simulink model "distmodelR2019a"  (R2020b)
settings: Solver=FixedStepAuto  StartTime=0.0  StopTime=t_sim  FixedStep=TimeStep  RelTol=1e-3
values from neighbouring files (symbols this model uses):
  alt = 300    [main_disturbances_Z.m]
  AX = 0.022    [calctorque.m]    (also in main_disturbances_Z.m)
  AY = 0.034    [calctorque.m]    (also in main_disturbances_Z.m)
  AZ = 0.0748    [calctorque.m]    (also in main_disturbances_Z.m = 0.2108)
  AZES = 0.1156    [calctorque.m]    (also in main_disturbances_Z.m)
  Cdrag = 2.6    [disturbanceCode.m]    (also in main_disturbances_Z.m)
  CLS = [0,-0.195,0.05]    [calctorque.m]    (also in main_disturbances_Z.m)
  Cmy = [0,-0.11,0]    [calctorque.m]    (also in main_disturbances_Z.m)
  CRS = [0,0.195,0.05]    [calctorque.m]    (also in main_disturbances_Z.m)
  D = [-0.17,0.11,0.05]    [projectionTorque1.m]    (also in projectionTorque2.m; projectionTorque3.m = [-0.17,-0.11,0.05]; projectionTorque4.m = [-0.17,-0.11,0.05])
  ESS = 0.0578    [calctorque.m]    (also in main_disturbances_Z.m)
  G = [OGX,OGY,OGZ]    [disturbanceCode.m]    (also in main_disturbances_Z.m)
  inc = rad2deg(inc)    [main_disturbances_Z.m]
  nu = rad2deg(nu)    [main_disturbances_Z.m]
  OGX = 2.5*1e-3    (= 0.0025)    [disturbanceCode.m]    (also in main_disturbances_Z.m = 0.00025)
  OGY = 1*1e-2    (= 0.01)    [disturbanceCode.m]    (also in main_disturbances_Z.m = -0.001)
  OGZ = 1*1e-2    (= 0.01)    [disturbanceCode.m]    (also in main_disturbances_Z.m = -0.002)
  OX = 0.17    [calctorque.m]    (also in main_disturbances_Z.m)
  OY = 0.11    [calctorque.m]    (also in main_disturbances_Z.m)
  OZ = 0.05    [calctorque.m]    (also in main_disturbances_Z.m)
  RAAN = rad2deg(RAAN)    [main_disturbances_Z.m]
  RSD = [0.08,0.08,0.08]    [main_disturbances_Z.m]
  w = rad2deg(w)    [main_disturbances_Z.m]
undefined symbols (not defined in the file or in its folder): date, DipoleMod, ecc, km, nmax, s, Use_IGRF
libraries: vrlib x19, dspmathops x6, sharedtransform x4, aerolibutil x4, dspindex x3, aerolibconvert2 x2, simulink_extras x1, aerolibatmos2 x1, aerolibcelestial x1, sharedutil x1, aerolibobsolete x1
(part 1 of 2)
settings Model: Creator=colpari  LastModifiedBy=colpari
settings SFSimCC: CustomCodeUndefinedFunction=UseInterfaceOnly

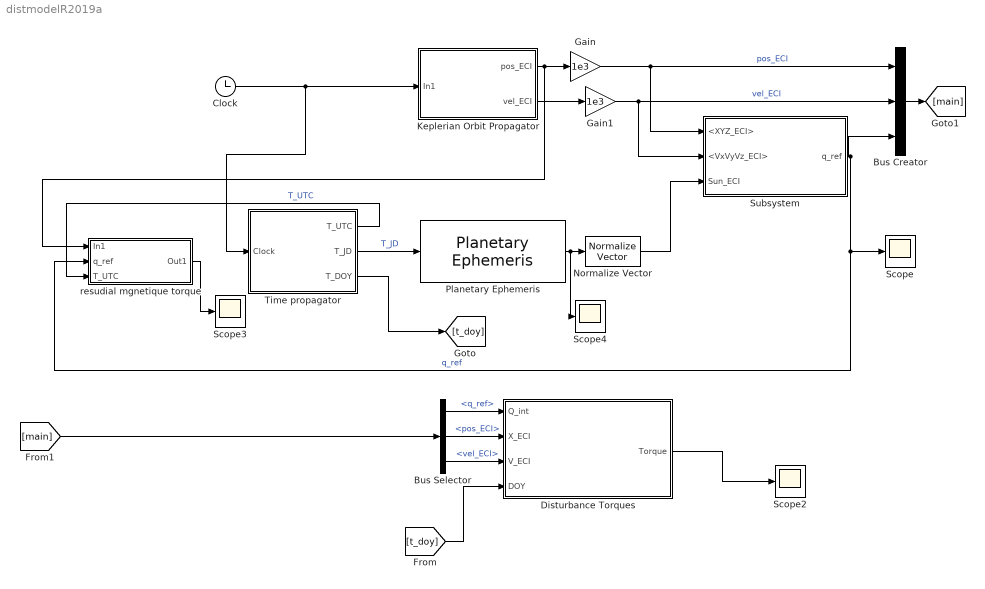
== system distmodelR2019a ==
  Bus Creator : BusCreator  Inputs=3
  Bus Selector : BusSelector  OutputSignals=q_ref,pos_ECI,vel_ECI
  Clock : Clock
  "Disturbance Torques " : Subsystem
  Gain : Gain  Gain=1e3
  Gain1 : Gain  Gain=1e3
  Keplerian Orbit Propagator : Subsystem
  Normalize Vector : vrlib/Utilities/Normalize Vector  maxzero=0
  Planetary Ephemeris : aerolibcelestial/Planetary Ephemeris  kmflag=km,km/s  epochflag=Julian date  de=DE405  nCenter=Earth  nTarget=Sun  errorflag=Error  velflag=off
      settings: SourceProductBaseCode=AE
  Scope{,2..4} (4 alike) : Scope
  Subsystem : Subsystem
  Time propagator : Subsystem
  "resudial mgnetique torque " : Subsystem
  wires:
  [t_doy] -> "Disturbance Torques "/4(DOY)
  "Disturbance Torques "/1("Torque ") -> Scope2/1
  Clock/1 -> Keplerian Orbit Propagator/1(In1), Time propagator/1(Clock)
  Keplerian Orbit Propagator/2(vel_ECI) -> Gain1/1
  Planetary Ephemeris/1 -> Scope4/1, Normalize Vector/1
  Normalize Vector/1 -> Subsystem/3(Sun_ECI)
  Time propagator/2(T_JD) -> Planetary Ephemeris/1  "T_JD"
  Subsystem/1(q_ref) -> Bus Creator/3, "resudial mgnetique torque "/2(q_ref), Scope/1  "q_ref"
  Time propagator/3(T_DOY) -> [t_doy]
  Bus Creator/1 -> [main]
  Time propagator/1(T_UTC) -> "resudial mgnetique torque "/3(T_UTC)  "T_UTC"
  [main] -> Bus Selector/1
  Gain/1 -> Subsystem/1(<XYZ_ECI>), Bus Creator/1  "pos_ECI"
  Gain1/1 -> Subsystem/2(<VxVyVz_ECI>), Bus Creator/2  "vel_ECI"
  Keplerian Orbit Propagator/1(pos_ECI) -> "resudial mgnetique torque "/1(In1), Gain/1
  "resudial mgnetique torque "/1(Out1) -> Scope3/1
  Bus Selector/1 -> "Disturbance Torques "/1("Q_int ")  "<q_ref>"
  Bus Selector/2 -> "Disturbance Torques "/2(X_ECI)  "<pos_ECI>"
  Bus Selector/3 -> "Disturbance Torques "/3(V_ECI)  "<vel_ECI>"

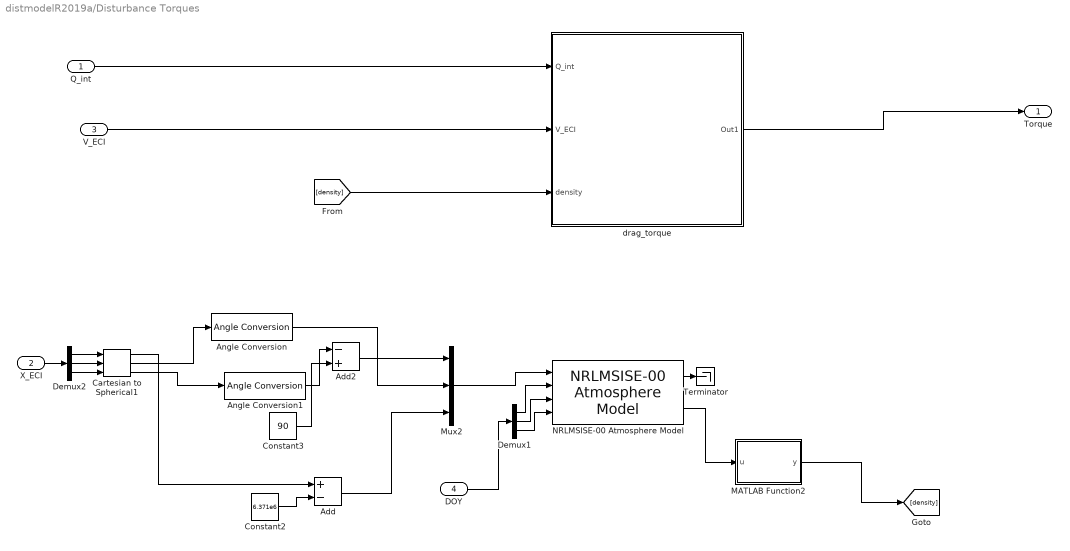
== system distmodelR2019a/Disturbance Torques  ==
  "Q_int " : Inport
  X_ECI : Inport  Port=2
  V_ECI : Inport  Port=3
  DOY : Inport  Port=4
  Add : Sum  Inputs=+-
  Add2 : Sum  Inputs=-+
  Angle Conversion : aerolibconvert2/Angle Conversion  IU=rad  OU=deg
  Angle Conversion1 : aerolibconvert2/Angle Conversion  IU=rad  OU=deg
  Cartesian to Spherical1 : simulink_extras/Transformations/Cartesian to Spherical
      settings: SourceProductBaseCode=SL
  Constant2 : Constant  Value=6.371e6
  Constant3 : Constant  Value=90
  Demux1 : Demux  Outputs=3
  Demux2 : Demux  Outputs=3
  MATLAB Function2 : MATLAB Function  TreatAsAtomicUnit=on
  Mux2 : Mux  Inputs=3
  NRLMSISE-00 Atmosphere Model : aerolibatmos2/NRLMSISE-00 Atmosphere Model  units=Metric (MKS)  lst_input=off  flux_ap_input=off  flags_input=Internal  flags=ones(1,23)  oxygen_in=on  action=Warning
      settings: SourceProductBaseCode=AE
  Terminator : Terminator
  drag_torque : Subsystem
  "Torque " : Outport
  wires:
  V_ECI/1 -> drag_torque/2(V_ECI)
  Demux1/1 -> NRLMSISE-00 Atmosphere Model/2
  Demux2/3 -> Cartesian to Spherical1/3
  Demux2/1 -> Cartesian to Spherical1/1
  Cartesian to Spherical1/1 -> Add/1
  Constant2/1 -> Add/2
  Demux2/2 -> Cartesian to Spherical1/2
  Demux1/2 -> NRLMSISE-00 Atmosphere Model/3
  NRLMSISE-00 Atmosphere Model/2 -> MATLAB Function2/1(u)
  MATLAB Function2/1(y) -> [density]
  Demux1/3 -> NRLMSISE-00 Atmosphere Model/4
  DOY/1 -> Demux1/1
  "Q_int "/1 -> drag_torque/1(Q_int)
  Mux2/1 -> NRLMSISE-00 Atmosphere Model/1
  Add/1 -> Mux2/3
  Cartesian to Spherical1/2 -> Angle Conversion/1
  Cartesian to Spherical1/3 -> Angle Conversion1/1
  Angle Conversion/1 -> Mux2/2
  Add2/1 -> Mux2/1
  Angle Conversion1/1 -> Add2/1
  Constant3/1 -> Add2/2
  NRLMSISE-00 Atmosphere Model/1 -> Terminator/1
  [density] -> drag_torque/3("density ")
  X_ECI/1 -> Demux2/1
  drag_torque/1(Out1) -> "Torque "/1

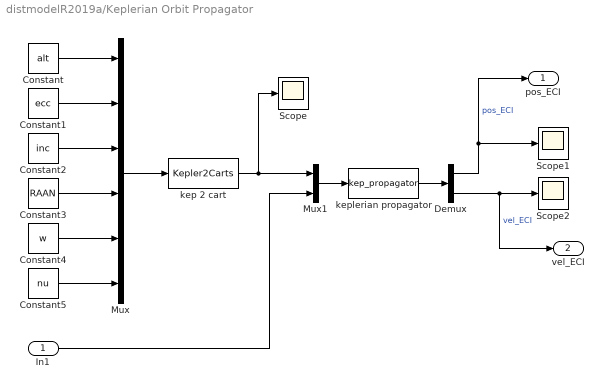
== system distmodelR2019a/Keplerian Orbit Propagator ==
  In1 : Inport
  Constant : Constant  Value=alt
  Constant1 : Constant  Value=ecc
  Constant2 : Constant  Value=inc
  Constant3 : Constant  Value=RAAN
  Constant4 : Constant  Value=w
  Constant5 : Constant  Value=nu
  Demux : Demux  Outputs=2
  Mux : Mux  Inputs=6
  Mux1 : Mux  Inputs=2
  Scope : Scope
  Scope1 : Scope
  Scope2 : Scope
  kep 2 cart : MATLABFcn  MATLABFcn=Kepler2Carts
  keplerian propagator : MATLABFcn  MATLABFcn=kep_propagator
  pos_ECI : Outport
  vel_ECI : Outport  Port=2
  wires:
  Mux/1 -> kep 2 cart/1
  Constant5/1 -> Mux/6
  Constant2/1 -> Mux/3
  kep 2 cart/1 -> Mux1/1, Scope/1
  Demux/2 -> vel_ECI/1, Scope2/1  "vel_ECI"
  Constant3/1 -> Mux/4
  Demux/1 -> pos_ECI/1, Scope1/1  "pos_ECI"
  Constant4/1 -> Mux/5
  keplerian propagator/1 -> Demux/1
  Mux1/1 -> keplerian propagator/1
  Constant/1 -> Mux/1
  Constant1/1 -> Mux/2
  In1/1 -> Mux1/2

== system distmodelR2019a/Subsystem ==
  <XYZ_ECI> : Inport
  <VxVyVz_ECI> : Inport  Port=2
  Sun_ECI : Inport  Port=3
  Manual Switch : ManualSwitch  CurrentSetting=0
  Terminator : Terminator
  q_orbital : Subsystem
  q_sun_aero : Subsystem
  q_sun_sun : Subsystem
  q_ref : Outport
  wires:
  q_sun_aero/1(Q_sun_aero) -> Manual Switch/2
  q_orbital/1(Q_orbit) -> Manual Switch/1
  <XYZ_ECI>/1 -> q_orbital/1(<XYZ_ECI>)
  Sun_ECI/1 -> q_sun_sun/2(GS_ECI), q_sun_aero/1(Sun_ECI)
  <VxVyVz_ECI>/1 -> q_sun_aero/2(<VxVyVz_ECI>), q_sun_sun/1(<VxVyVz_ECI>), q_orbital/2(<VxVyVz_ECI>)
  Manual Switch/1 -> q_ref/1
  q_sun_sun/1(Q_sun_sun) -> Terminator/1

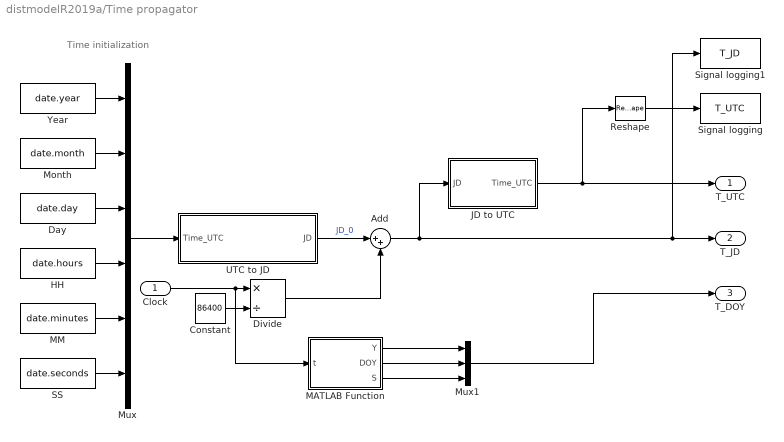
== system distmodelR2019a/Time propagator ==
  note: Time initialization
  Clock : Inport
  Add : Sum  Inputs=|++
  Constant : Constant  Value=86400
  Day : Constant  Value=date.day
  Divide : Product  Inputs=*/
  HH : Constant  Value=date.hours
  JD to UTC : MATLAB Function  TreatAsAtomicUnit=on
  MATLAB Function : MATLAB Function  TreatAsAtomicUnit=on
  MM : Constant  Value=date.minutes
  Month : Constant  Value=date.month
  Mux : Mux  Inputs=6
  Mux1 : Mux  Inputs=3
  Reshape : Reshape
  SS : Constant  Value=date.seconds
  Signal logging : ToWorkspace  VariableName=T_UTC  SaveFormat=Timeseries  SampleTime=1
      settings: Save2DSignal=2-D array (concatenate along first dimension)
  Signal logging1 : ToWorkspace  VariableName=T_JD  SaveFormat=Timeseries  SampleTime=1
      settings: Save2DSignal=2-D array (concatenate along first dimension)
  UTC to JD : MATLAB Function  TreatAsAtomicUnit=on
  Year : Constant  Value=date.year
  T_UTC : Outport  VectorParamsAs1DForOutWhenUnconnected=off
  T_JD : Outport  Port=2  VectorParamsAs1DForOutWhenUnconnected=off
  T_DOY : Outport  Port=3
  wires:
  UTC to JD/1(JD) -> Add/1  "JD_0"
  Clock/1 -> MATLAB Function/1(t), Divide/1
  Constant/1 -> Divide/2
  JD to UTC/1(Time_UTC) -> T_UTC/1, Reshape/1
  Divide/1 -> Add/2
  Mux/1 -> UTC to JD/1(Time_UTC)
  Day/1 -> Mux/3
  Month/1 -> Mux/2
  Year/1 -> Mux/1
  HH/1 -> Mux/4
  MM/1 -> Mux/5
  SS/1 -> Mux/6
  Reshape/1 -> Signal logging/1
  Add/1 -> Signal logging1/1, T_JD/1, JD to UTC/1(JD)
  MATLAB Function/1(Y) -> Mux1/1
  MATLAB Function/2(DOY) -> Mux1/2
  MATLAB Function/3(S) -> Mux1/3
  Mux1/1 -> T_DOY/1

== system distmodelR2019a/resudial mgnetique torque  ==
  In1 : Inport
  q_ref : Inport  Port=2
  T_UTC : Inport  Port=3
  Constant : Constant  Value=RSD
  Cross Product : vrlib/Utilities/Cross Product
  DCMi2e : Subsystem  TreatAsAtomicUnit=on  SystemSampleTime=1
  IGRF Computation block : Subsystem
  Reshape : Reshape  OutputDimensionality=Column vector (2-D)
  Reshape1 : Reshape  OutputDimensionality=Column vector (2-D)
  Scope : Scope
  Subsystem1 : Subsystem
  Out1 : Outport  VectorParamsAs1DForOutWhenUnconnected=off
  wires:
  In1/1 -> IGRF Computation block/1(<XYZ_ECI>)
  T_UTC/1 -> DCMi2e/1(Time_UTC), IGRF Computation block/3("Time_UTC ")
  IGRF Computation block/1(B_ECI) -> Subsystem1/2(B_ECI)
  q_ref/1 -> Subsystem1/1(<Q_ECI>)
  DCMi2e/1(DCM_i2e) -> IGRF Computation block/2("DCM_i2e ")
  Constant/1 -> Reshape/1
  Subsystem1/1(B_body) -> Reshape1/1
  Reshape/1 -> Cross Product/1
  Reshape1/1 -> Cross Product/2
  Cross Product/1 -> Scope/1, Out1/1

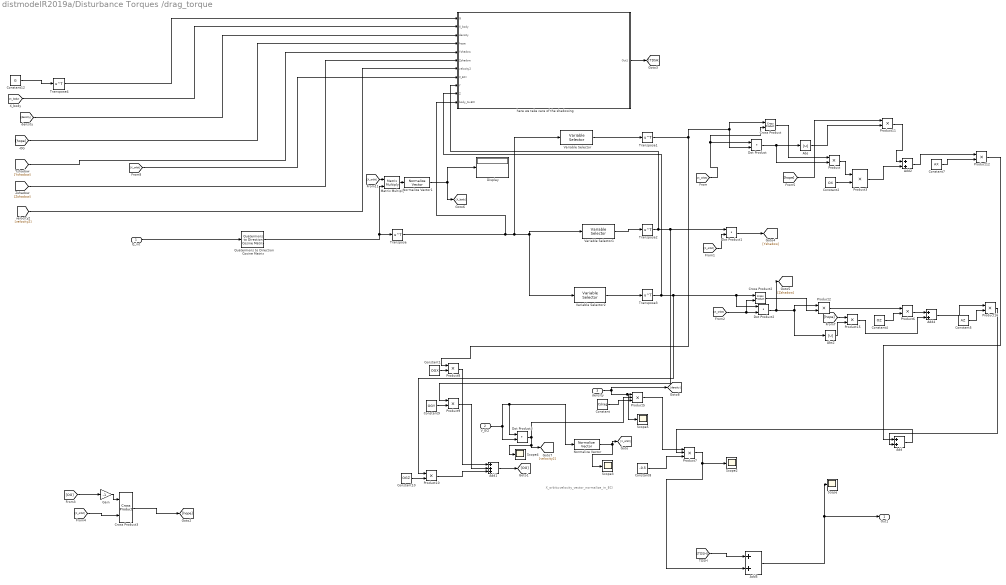
== system distmodelR2019a/Disturbance Torques /drag_torque ==
  note: X_orbit=velocity_vector_normalize_in_ECI
  Q_int : Inport
  V_ECI : Inport  Port=2
  "density " : Inport  Port=3
  Abs : Abs
  Abs2 : Abs
  Add{,2,4..5} (4 alike) : Sum
  Add1 : Sum  Inputs=+++
  Constant : Constant  Value=Cdrag
  Constant1 : Constant  Value=OGX
  Constant10 : Constant  Value=OGZ
  Constant12 : Constant  Value=G
  Constant2 : Constant  Value=OX
  Constant4 : Constant  Value=OZ
  Constant5 : Constant  Value=AZ
  Constant7 : Constant  Value=AX
  Constant8 : Constant  Value=-0.5
  Constant9 : Constant  Value=OGY
  Cross Product : vrlib/Utilities/Cross Product
  Cross Product2 : vrlib/Utilities/Cross Product
  Cross Product3 : vrlib/Utilities/Cross Product
  Display : Display
  Dot Product{,1..3} (4 alike) : DotProduct  InputSameDT=on  OutDataTypeStr=Inherit: Inherit via internal rule
  Gain : Gain  Gain=-1
  Matrix Multiply : Product  Multiplication=Matrix(*)
  Normalize Vector : vrlib/Utilities/Normalize Vector  maxzero=0
  Normalize Vector1 : vrlib/Utilities/Normalize Vector  maxzero=0
  Product{,2..3,6,8..12,15..16} (11 alike) : Product
  Product5 : Product  Inputs=3
  Product7 : Product  Inputs=3
  Quaternions to Direction Cosine Matrix : sharedtransform/Quaternions to  Direction Cosine Matrix  aMode=aMode
      settings: SourceProductBaseCode=AE,PW,MT,UV,VE,VP
  Scope{,2..5} (5 alike) : Scope
  Transpose{,1..4} (5 alike) : Math  Operator=transpose  SignedPower=on  SaturateOnIntegerOverflow=on
  Variable Selector : dspindex/Variable Selector  NumInputs=1  rowsOrCols=Columns  IdxMode=Fixed  Elements=[1]  ZerOneIdxMode=One-based  errmode=Clip Index  FillMode=on  FillValues=0
  Variable Selector1 : dspindex/Variable Selector  NumInputs=1  rowsOrCols=Columns  IdxMode=Fixed  Elements=[2]  ZerOneIdxMode=One-based  errmode=Clip Index  FillMode=on  FillValues=0
  Variable Selector2 : dspindex/Variable Selector  NumInputs=1  rowsOrCols=Columns  IdxMode=Fixed  Elements=[3]  ZerOneIdxMode=One-based  errmode=Clip Index  FillMode=on  FillValues=0
  "here we take care of the shadowing " : Subsystem
  Out1 : Outport  VectorParamsAs1DForOutWhenUnconnected=off
  wires:
  Quaternions to Direction Cosine Matrix/1 -> Matrix Multiply/2, Transpose/1
  Q_int/1 -> Quaternions to Direction Cosine Matrix/1
  Normalize Vector/1 -> [X_orbit], Scope3/1
  [X_orbit] -> Cross Product/2, Dot Product/1
  [X_orbit] -> Dot Product2/2, Cross Product2/2
  Cross Product/1 -> Product/1
  Cross Product2/1 -> Product2/2
  Dot Product2/1 -> [Zshadow], Abs2/1, Product2/1
  Constant2/1 -> Product3/2
  Constant4/1 -> Product6/2
  Constant/1 -> Product5/3
  Product5/1 -> Product7/1
  Add/1 -> Product7/2
  Constant8/1 -> Product7/3
  Product7/1 -> Scope2/1, Add5/2
  Dot Product3/1 -> Scope4/1, [velocity2], Product5/2
  Dot Product/1 -> Product/2, Abs/1
  Variable Selector/1 -> Transpose1/1
  Variable Selector1/1 -> Transpose2/1
  Variable Selector2/1 -> Transpose3/1
  Constant1/1 -> Product8/2
  Constant9/1 -> Product9/2
  Constant10/1 -> Product10/2
  Product10/1 -> Add1/3
  Product9/1 -> Add1/2
  Product8/1 -> Add1/1
  Add1/1 -> [OG]
  Gain/1 -> Cross Product3/1
  [OG] -> Gain/1
  [X_orbit] -> Cross Product3/2
  Product/1 -> Product3/1
  Cross Product3/1 -> [hope]
  Abs/1 -> Product11/2
  [hope] -> Product11/1
  Product11/1 -> Add2/1
  Product3/1 -> Add2/2
  Add2/1 -> Product12/1
  Constant7/1 -> Product12/2
  Product12/1 -> Add/1
  Abs2/1 -> Product15/2
  [hope] -> Product15/1
  Product2/1 -> Product6/1
  Product6/1 -> Add4/1
  Product15/1 -> Add4/2
  Add4/1 -> Product16/1
  Constant5/1 -> Product16/2
  [X_orbit] -> Matrix Multiply/1
  Constant12/1 -> Transpose4/1
  "density "/1 -> [density], Scope5/1, Product5/1
  V_ECI/1 -> Normalize Vector/1, Dot Product3/1, Dot Product3/2
  Transpose2/1 -> "here we take care of the shadowing "/9(Y), Dot Product1/1, Product9/1
  Add5/1 -> Scope/1, Out1/1
  Product16/1 -> Add/2
  Matrix Multiply/1 -> Normalize Vector1/1
  Normalize Vector1/1 -> [X_body], Display/1
  Transpose4/1 -> "here we take care of the shadowing "/1(G)
  [X_body] -> "here we take care of the shadowing "/2(X_body)
  [density] -> "here we take care of the shadowing "/3(density)
  [hope] -> "here we take care of the shadowing "/4(hope)
  [Yshadow] -> "here we take care of the shadowing "/5(Yshadow)
  [Zshadow] -> "here we take care of the shadowing "/6(Zshadow)
  [velocity2] -> "here we take care of the shadowing "/7(velocity2)
  [X_orbit] -> "here we take care of the shadowing "/8(V_ECI)
  Transpose/1 -> "here we take care of the shadowing "/11(body_to-ECI), Variable Selector2/1, Variable Selector1/1, Variable Selector/1
  Transpose3/1 -> Product10/1, Dot Product2/1, Cross Product2/1, "here we take care of the shadowing "/10(Z)
  Transpose1/1 -> Product8/1, Dot Product/2, Cross Product/1
  "here we take care of the shadowing "/1(Out1) -> [TDSH]
  [TDSH] -> Add5/1
  [X_orbit] -> Dot Product1/2
  Dot Product1/1 -> [Yshadow]

== system distmodelR2019a/Subsystem/q_orbital ==
  <XYZ_ECI> : Inport
  <VxVyVz_ECI> : Inport  Port=2
  3x3 Cross Product : sharedutil/3x3 Cross Product  aMode=aMode
      settings: SourceProductBaseCode=AE,PW,MT,UV,VE,VP
  Direction Cosine Matrix to Quaternions : sharedtransform/Direction Cosine Matrix  to Quaternions  aMode=0  action=None  tolerance=eps(2)
      settings: SourceProductBaseCode=AE,PW,MT,UV,VE,VP
  Gain : Gain
  Gain1 : Gain  Gain=-1
  Normalization : dspmathops/Normalization  NormType=2-norm  Bias=1e-10  NormOver=Each column  Dimension=1  roundingMode=Floor  overflowMode=off  accumDataTypeStr=Inherit: Same as product output  accumLastDataTypeStr=Inherit: Same as product output  outputDataTypeStr=Inherit: Same as product output  outputMin=[]  outputMax=[]  outputLastDataTypeStr=Inherit: Same as product output
  Normalization1 : dspmathops/Normalization  NormType=2-norm  Bias=1e-10  NormOver=Each column  Dimension=1  roundingMode=Floor  overflowMode=off  accumDataTypeStr=Inherit: Same as product output  accumLastDataTypeStr=Inherit: Same as product output  outputDataTypeStr=Inherit: Same as product output  outputMin=[]  outputMax=[]  outputLastDataTypeStr=Inherit: Same as product output
  Quaternion Inverse : aerolibutil/Quaternion Inverse
  Reshape : Reshape  OutputDimensionality=Column vector (2-D)
  Reshape1 : Reshape  OutputDimensionality=Column vector (2-D)
  Vector Concatenate : Concatenate  NumInputs=3  Mode=Multidimensional array  ConcatenateDimension=2
  Q_orbit : Outport  VectorParamsAs1DForOutWhenUnconnected=off
  wires:
  Normalization/1 -> Reshape/1
  Normalization1/1 -> Reshape1/1
  <VxVyVz_ECI>/1 -> Normalization1/1
  Reshape1/1 -> 3x3 Cross Product/1, Vector Concatenate/1
  <XYZ_ECI>/1 -> Normalization/1
  Reshape/1 -> Gain/1
  Gain/1 -> 3x3 Cross Product/2, Vector Concatenate/3
  Direction Cosine Matrix to Quaternions/1 -> Quaternion Inverse/1
  3x3 Cross Product/1 -> Gain1/1
  Gain1/1 -> Vector Concatenate/2
  Quaternion Inverse/1 -> Q_orbit/1
  Vector Concatenate/1 -> Direction Cosine Matrix to Quaternions/1

== system distmodelR2019a/Subsystem/q_sun_aero ==
  note: choix :
      | x selon V
      | z tel que z.GS soit maximisé
  Sun_ECI : Inport
  <VxVyVz_ECI> : Inport  Port=2
  Cross Product : vrlib/Utilities/Cross Product
  Direction Cosine Matrix to Quaternions : sharedtransform/Direction Cosine Matrix  to Quaternions  aMode=0  action=None  tolerance=eps(2)
      settings: SourceProductBaseCode=AE,PW,MT,UV,VE,VP
  Dot Product : DotProduct  InputSameDT=on  OutDataTypeStr=Inherit: Inherit via internal rule
  Normalization1 : dspmathops/Normalization  NormType=2-norm  Bias=1e-10  NormOver=Each column  Dimension=1  roundingMode=Floor  overflowMode=off  accumDataTypeStr=Inherit: Same as product output  accumLastDataTypeStr=Inherit: Same as product output  outputDataTypeStr=Inherit: Same as product output  outputMin=[]  outputMax=[]  outputLastDataTypeStr=Inherit: Same as product output
  Normalization2 : dspmathops/Normalization  NormType=2-norm  Bias=1e-10  NormOver=Each column  Dimension=1  roundingMode=Floor  overflowMode=off  accumDataTypeStr=Inherit: Same as product output  accumLastDataTypeStr=Inherit: Same as product output  outputDataTypeStr=Inherit: Same as product output  outputMin=[]  outputMax=[]  outputLastDataTypeStr=Inherit: Same as product output
  Plus : Sum  Inputs=-+
  Product : Product
  Quaternion Inverse : aerolibutil/Quaternion Inverse
  Reshape1 : Reshape  OutputDimensionality=Column vector (2-D)
  Reshape2 : Reshape  OutputDimensionality=Column vector (2-D)
  Reshape3 : Reshape  OutputDimensionality=Column vector (2-D)
  Vector Concatenate : Concatenate  NumInputs=3  Mode=Multidimensional array  ConcatenateDimension=2
  Q_sun_aero : Outport  VectorParamsAs1DForOutWhenUnconnected=off
  wires:
  Quaternion Inverse/1 -> Q_sun_aero/1
  Reshape2/1 -> Vector Concatenate/3, Cross Product/1
  Reshape3/1 -> Vector Concatenate/1, Cross Product/2
  Product/1 -> Plus/1
  Dot Product/1 -> Product/2
  Cross Product/1 -> Reshape1/1  "y"
  Normalization2/1 -> Reshape2/1  "z"
  Plus/1 -> Normalization2/1  "GS-(GS.x)x"
  Sun_ECI/1 -> Dot Product/2, Plus/2
  Vector Concatenate/1 -> Direction Cosine Matrix to Quaternions/1
  Direction Cosine Matrix to Quaternions/1 -> Quaternion Inverse/1
  Normalization1/1 -> Dot Product/1, Product/1, Reshape3/1  "x"
  <VxVyVz_ECI>/1 -> Normalization1/1
  Reshape1/1 -> Vector Concatenate/2

== system distmodelR2019a/Subsystem/q_sun_sun ==
  note: Choix:
      | z selon GS
      | x tel que x.V soit maximisé
  <VxVyVz_ECI> : Inport
  GS_ECI : Inport  Port=2
  Cross Product1 : vrlib/Utilities/Cross Product
  Direction Cosine Matrix to Quaternions1 : sharedtransform/Direction Cosine Matrix  to Quaternions  aMode=0  action=None  tolerance=eps(2)
      settings: SourceProductBaseCode=AE,PW,MT,UV,VE,VP
  Dot Product1 : DotProduct  InputSameDT=on  OutDataTypeStr=Inherit: Inherit via internal rule
  Normalization3 : dspmathops/Normalization  NormType=2-norm  Bias=1e-10  NormOver=Each column  Dimension=1  roundingMode=Floor  overflowMode=off  accumDataTypeStr=Inherit: Same as product output  accumLastDataTypeStr=Inherit: Same as product output  outputDataTypeStr=Inherit: Same as product output  outputMin=[]  outputMax=[]  outputLastDataTypeStr=Inherit: Same as product output
  Normalization4 : dspmathops/Normalization  NormType=2-norm  Bias=1e-10  NormOver=Each column  Dimension=1  roundingMode=Floor  overflowMode=off  accumDataTypeStr=Inherit: Same as product output  accumLastDataTypeStr=Inherit: Same as product output  outputDataTypeStr=Inherit: Same as product output  outputMin=[]  outputMax=[]  outputLastDataTypeStr=Inherit: Same as product output
  Plus1 : Sum  Inputs=-+
  Product1 : Product
  Quaternion Inverse1 : aerolibutil/Quaternion Inverse
  Reshape4 : Reshape  OutputDimensionality=Column vector (2-D)
  Reshape5 : Reshape  OutputDimensionality=Column vector (2-D)
  Reshape6 : Reshape  OutputDimensionality=Column vector (2-D)
  Vector Concatenate1 : Concatenate  NumInputs=3  Mode=Multidimensional array  ConcatenateDimension=2
  Q_sun_sun : Outport  VectorParamsAs1DForOutWhenUnconnected=off
  wires:
  Quaternion Inverse1/1 -> Q_sun_sun/1
  Dot Product1/1 -> Product1/1
  Reshape6/1 -> Cross Product1/1, Vector Concatenate1/3
  Reshape5/1 -> Cross Product1/2, Vector Concatenate1/1
  <VxVyVz_ECI>/1 -> Dot Product1/1, Plus1/1
  GS_ECI/1 -> Normalization3/1
  Vector Concatenate1/1 -> Direction Cosine Matrix to Quaternions1/1
  Product1/1 -> Plus1/2
  Plus1/1 -> Normalization4/1  "V-(V.z)z"
  Cross Product1/1 -> Reshape4/1  "y"
  Normalization4/1 -> Reshape5/1  "x"
  Normalization3/1 -> Dot Product1/2, Product1/2, Reshape6/1  "z"
  Direction Cosine Matrix to Quaternions1/1 -> Quaternion Inverse1/1
  Reshape4/1 -> Vector Concatenate1/2

== system distmodelR2019a/resudial mgnetique torque /DCMi2e ==
  note: Slower subsytem because it's too slow
  Time_UTC : Inport
  ECI to ECEF : MATLABFcn  MATLABFcn=eci2ecef  OutputDimensions=[3;3]  Output1D=off
  DCM_i2e : Outport
  wires:
  ECI to ECEF/1 -> DCM_i2e/1
  Time_UTC/1 -> ECI to ECEF/1

== system distmodelR2019a/resudial mgnetique torque /IGRF Computation block ==
  <XYZ_ECI> : Inport
  "DCM_i2e " : Inport  Port=2
  "Time_UTC " : Inport  Port=3
  Bus Creator : BusCreator  Inputs=5
  Demux : Demux  Outputs=2
  ECI To LLA : MATLAB Function  TreatAsAtomicUnit=on
  Obtain B_ECI : Subsystem
  Product : Product  Multiplication=Matrix(*)
  Reshape : Reshape  OutputDimensionality=Row vector (2-D)
  Terminator : Terminator
  B_ECI : Outport  VectorParamsAs1DForOutWhenUnconnected=off
  wires:
  ECI To LLA/3(long) -> Bus Creator/3
  ECI To LLA/2(lat) -> Bus Creator/2
  ECI To LLA/1(h) -> Bus Creator/1
  Demux/1 -> Bus Creator/4
  Demux/2 -> Terminator/1
  "DCM_i2e "/1 -> Product/2, Bus Creator/5  "DCM_i2e"
  Reshape/1 -> Product/1
  Product/1 -> ECI To LLA/1(X_ECEF)
  <XYZ_ECI>/1 -> Reshape/1
  "Time_UTC "/1 -> Demux/1
  Obtain B_ECI/1(Out1) -> B_ECI/1
  Bus Creator/1 -> Obtain B_ECI/1(In1)

== system distmodelR2019a/resudial mgnetique torque /Subsystem1 ==
  <Q_ECI> : Inport
  B_ECI : Inport  Port=2
  Quaternion Rotation : aerolibutil/Quaternion Rotation
  B_body : Outport
  wires:
  <Q_ECI>/1 -> Quaternion Rotation/1
  B_ECI/1 -> Quaternion Rotation/2
  Quaternion Rotation/1 -> B_body/1  "B_IGRF_body"

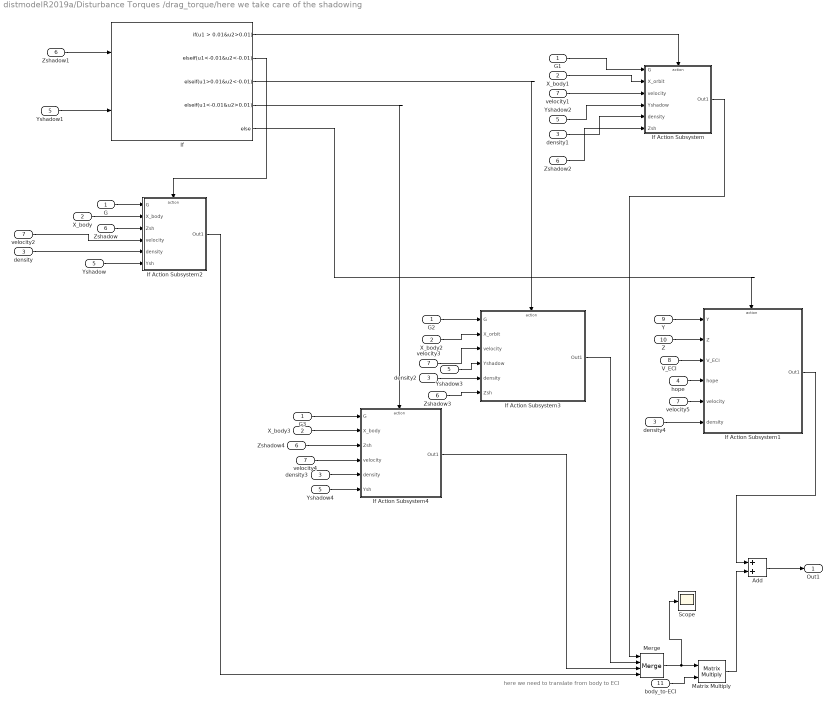
== system distmodelR2019a/Disturbance Torques /drag_torque/here we take care of the shadowing  ==
  note: here we need to translate from body to ECI
  G : Inport
  X_body : Inport  Port=2
  density : Inport  Port=3
  hope : Inport  Port=4
  Yshadow : Inport  Port=5
  Zshadow : Inport  Port=6
  velocity2 : Inport  Port=7
  V_ECI : Inport  Port=8
  Y : Inport  Port=9
  Z : Inport  Port=10
  body_to-ECI : Inport  Port=11
  Add : Sum
  G1 : InportShadow
  G2 : InportShadow
  G3 : InportShadow
  If : If  NumInputs=2  IfExpression=u1 > 0.01&u2>0.01  ElseIfExpressions=u1<-0.01&u2<-0.01,u1>0.01&u2<-0.01,u1<-0.01&u2>0.01
  If Action Subsystem : Subsystem  TreatAsAtomicUnit=on
  If Action Subsystem1 : Subsystem  TreatAsAtomicUnit=on
  If Action Subsystem2 : Subsystem  TreatAsAtomicUnit=on
  If Action Subsystem3 : Subsystem  TreatAsAtomicUnit=on
  If Action Subsystem4 : Subsystem  TreatAsAtomicUnit=on
  Matrix Multiply : Product  Multiplication=Matrix(*)
  Merge : Merge  Inputs=4
  Scope : Scope
  X_body1 : InportShadow  Port=2
  X_body2 : InportShadow  Port=2
  X_body3 : InportShadow  Port=2
  Yshadow{1..4} (4 alike) : InportShadow  Port=5
  Zshadow{1..4} (4 alike) : InportShadow  Port=6
  density{1..4} (4 alike) : InportShadow  Port=3
  velocity{1,3..5} (4 alike) : InportShadow  Port=7
  Out1 : Outport  VectorParamsAs1DForOutWhenUnconnected=off
  wires:
  If/2 -> If Action Subsystem2/Action
  If/1 -> If Action Subsystem/Action
  If Action Subsystem4/1(Out1) -> Merge/3
  If/5 -> If Action Subsystem1/Action
  If/3 -> If Action Subsystem3/Action
  If Action Subsystem/1(Out1) -> Merge/1
  If Action Subsystem3/1(Out1) -> Merge/2
  If/4 -> If Action Subsystem4/Action
  If Action Subsystem2/1(Out1) -> Merge/4
  G1/1 -> If Action Subsystem/1(G)
  G/1 -> If Action Subsystem2/1(G)
  Zshadow1/1 -> If/1
  Yshadow1/1 -> If/2
  density/1 -> If Action Subsystem2/5(density)
  velocity2/1 -> If Action Subsystem2/4(velocity)
  X_body/1 -> If Action Subsystem2/2(X_body)
  Zshadow/1 -> If Action Subsystem2/3(Zsh)
  Yshadow/1 -> If Action Subsystem2/6(Ysh)
  X_body1/1 -> If Action Subsystem/2(X_orbit)
  Zshadow2/1 -> If Action Subsystem/6("Zsh ")
  velocity1/1 -> If Action Subsystem/3(velocity)
  Yshadow2/1 -> If Action Subsystem/4(Yshadow)
  density1/1 -> If Action Subsystem/5(density)
  G2/1 -> If Action Subsystem3/1(G)
  X_body2/1 -> If Action Subsystem3/2(X_orbit)
  velocity3/1 -> If Action Subsystem3/3(velocity)
  density2/1 -> If Action Subsystem3/5(density)
  Yshadow3/1 -> If Action Subsystem3/4(Yshadow)
  Zshadow3/1 -> If Action Subsystem3/6(Zsh)
  X_body3/1 -> If Action Subsystem4/2(X_body)
  G3/1 -> If Action Subsystem4/1(G)
  Yshadow4/1 -> If Action Subsystem4/6(Ysh)
  Zshadow4/1 -> If Action Subsystem4/3(Zsh)
  velocity4/1 -> If Action Subsystem4/4(velocity)
  density3/1 -> If Action Subsystem4/5(density)
  hope/1 -> If Action Subsystem1/4(hope)
  V_ECI/1 -> If Action Subsystem1/3(V_ECI)
  velocity5/1 -> If Action Subsystem1/5(velocity)
  density4/1 -> If Action Subsystem1/6(density)
  Z/1 -> If Action Subsystem1/2("Z ")
  Y/1 -> If Action Subsystem1/1(Y)
  Merge/1 -> Scope/1, Matrix Multiply/1
  body_to-ECI/1 -> Matrix Multiply/2
  If Action Subsystem1/1(Out1) -> Add/1
  Matrix Multiply/1 -> Add/2
  Add/1 -> Out1/1

== system distmodelR2019a/resudial mgnetique torque /IGRF Computation block/Obtain B_ECI ==
  In1 : Inport
  Dipole Subsystem : Subsystem  TreatAsAtomicUnit=on
  IGRF Subsystem : Subsystem  TreatAsAtomicUnit=on
  If : If
  Merge : Merge
  Use_IGRF : Constant  Value=Use_IGRF
  Out1 : Outport  VectorParamsAs1DForOutWhenUnconnected=off
  wires:
  If/1 -> IGRF Subsystem/Action
  In1/1 -> Dipole Subsystem/1(In1), IGRF Subsystem/1(In1)
  IGRF Subsystem/1(Out1) -> Merge/1
  Use_IGRF/1 -> If/1
  Merge/1 -> Out1/1
  Dipole Subsystem/1("B_ECI ") -> Merge/2
  If/2 -> Dipole Subsystem/Action

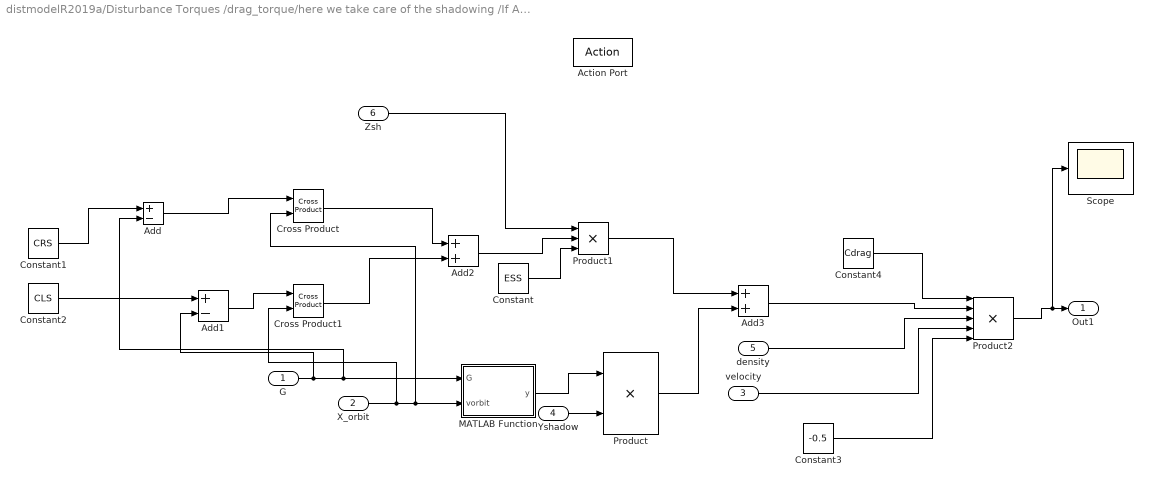
== system distmodelR2019a/Disturbance Torques /drag_torque/here we take care of the shadowing /If Action Subsystem ==
  G : Inport
  X_orbit : Inport  Port=2
  velocity : Inport  Port=3
  Yshadow : Inport  Port=4
  density : Inport  Port=5
  "Zsh " : Inport  Port=6
  Action Port : ActionPort  ActionPortLabel=if(u1 > 0.01&u2>0.01)
  Add : Sum  Inputs=+-
  Add1 : Sum  Inputs=+-
  Add2 : Sum
  Add3 : Sum
  Constant : Constant  Value=ESS
  Constant1 : Constant  Value=CRS
  Constant2 : Constant  Value=CLS
  Constant3 : Constant  Value=-0.5
  Constant4 : Constant  Value=Cdrag
  Cross Product : vrlib/Utilities/Cross Product
  Cross Product1 : vrlib/Utilities/Cross Product
  MATLAB Function : MATLAB Function  TreatAsAtomicUnit=on
  Product : Product
  Product1 : Product  Inputs=3
  Product2 : Product  Inputs=5
  Scope : Scope
  Out1 : Outport  VectorParamsAs1DForOutWhenUnconnected=off
  wires:
  G/1 -> Add1/2, Add/2, MATLAB Function/1(G)
  MATLAB Function/1(y) -> Product/1
  Yshadow/1 -> Product/2
  X_orbit/1 -> Cross Product1/2, Cross Product/2, MATLAB Function/2(vorbit)
  Constant1/1 -> Add/1
  Add/1 -> Cross Product/1
  Constant2/1 -> Add1/1
  Add1/1 -> Cross Product1/1
  Cross Product/1 -> Add2/1
  Cross Product1/1 -> Add2/2
  "Zsh "/1 -> Product1/1
  Add2/1 -> Product1/2
  Constant/1 -> Product1/3
  Product/1 -> Add3/2
  Product1/1 -> Add3/1
  Add3/1 -> Product2/2
  density/1 -> Product2/3
  velocity/1 -> Product2/4
  Product2/1 -> Scope/1, Out1/1
  Constant3/1 -> Product2/5
  Constant4/1 -> Product2/1

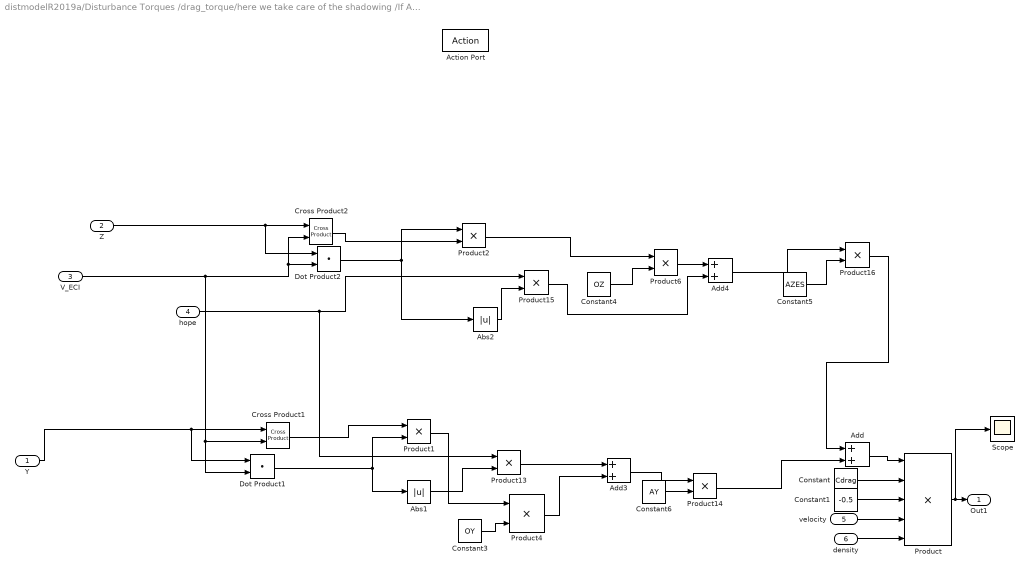
== system distmodelR2019a/Disturbance Torques /drag_torque/here we take care of the shadowing /If Action Subsystem1 ==
  Y : Inport
  "Z " : Inport  Port=2
  V_ECI : Inport  Port=3
  hope : Inport  Port=4
  velocity : Inport  Port=5
  density : Inport  Port=6
  Action Port : ActionPort  ActionPortLabel=else
  Abs1 : Abs
  Abs2 : Abs
  Add : Sum
  Add3 : Sum
  Add4 : Sum
  Constant : Constant  Value=Cdrag
  Constant1 : Constant  Value=-0.5
  Constant3 : Constant  Value=OY
  Constant4 : Constant  Value=OZ
  Constant5 : Constant  Value=AZES
  Constant6 : Constant  Value=AY
  Cross Product1 : vrlib/Utilities/Cross Product
  Cross Product2 : vrlib/Utilities/Cross Product
  Dot Product1 : DotProduct  InputSameDT=on  OutDataTypeStr=Inherit: Inherit via internal rule
  Dot Product2 : DotProduct  InputSameDT=on  OutDataTypeStr=Inherit: Inherit via internal rule
  Product : Product  Inputs=5
  Product{1..2,4,6,13..16} (8 alike) : Product
  Scope : Scope
  Out1 : Outport  VectorParamsAs1DForOutWhenUnconnected=off
  wires:
  Cross Product2/1 -> Product2/2
  Product15/1 -> Add4/2
  Add4/1 -> Product16/1
  Constant5/1 -> Product16/2
  Product6/1 -> Add4/1
  Abs2/1 -> Product15/2
  Product2/1 -> Product6/1
  Constant4/1 -> Product6/2
  "Z "/1 -> Dot Product2/1, Cross Product2/1
  Dot Product2/1 -> Abs2/1, Product2/1
  hope/1 -> Product13/1, Product15/1
  Product4/1 -> Add3/2
  Cross Product1/1 -> Product1/1
  Add3/1 -> Product14/1
  Product1/1 -> Product4/1
  Product13/1 -> Add3/1
  Y/1 -> Dot Product1/1, Cross Product1/1
  Abs1/1 -> Product13/2
  V_ECI/1 -> Dot Product1/2, Cross Product1/2, Dot Product2/2, Cross Product2/2
  Constant6/1 -> Product14/2
  Dot Product1/1 -> Abs1/1, Product1/2
  Constant3/1 -> Product4/2
  Product16/1 -> Add/1
  Product14/1 -> Add/2
  Add/1 -> Product/1
  Constant/1 -> Product/2
  Constant1/1 -> Product/3
  velocity/1 -> Product/4
  density/1 -> Product/5
  Product/1 -> Scope/1, Out1/1

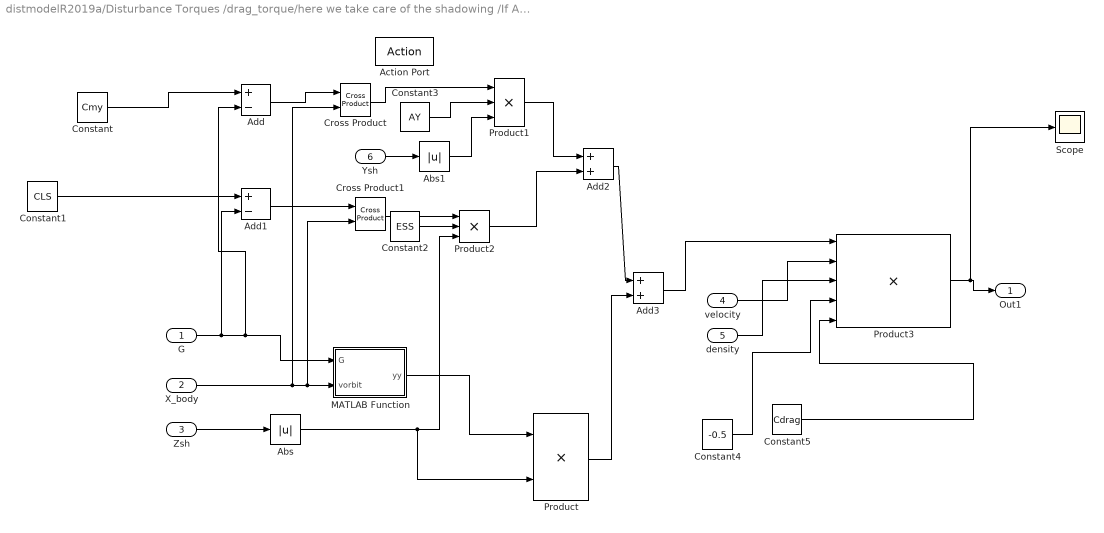
== system distmodelR2019a/Disturbance Torques /drag_torque/here we take care of the shadowing /If Action Subsystem2 ==
  G : Inport
  X_body : Inport  Port=2
  Zsh : Inport  Port=3
  velocity : Inport  Port=4
  density : Inport  Port=5
  Ysh : Inport  Port=6
  Action Port : ActionPort  ActionPortLabel=elseif(u1<-0.01&u2<-0.01)
  Abs : Abs
  Abs1 : Abs
  Add : Sum  Inputs=+-
  Add1 : Sum  Inputs=+-
  Add2 : Sum
  Add3 : Sum
  Constant : Constant  Value=Cmy
  Constant1 : Constant  Value=CLS
  Constant2 : Constant  Value=ESS
  Constant3 : Constant  Value=AY
  Constant4 : Constant  Value=-0.5
  Constant5 : Constant  Value=Cdrag
  Cross Product : vrlib/Utilities/Cross Product
  Cross Product1 : vrlib/Utilities/Cross Product
  MATLAB Function : MATLAB Function  TreatAsAtomicUnit=on
  Product : Product
  Product1 : Product  Inputs=3
  Product2 : Product  Inputs=3
  Product3 : Product  Inputs=5
  Scope : Scope
  Out1 : Outport  VectorParamsAs1DForOutWhenUnconnected=off
  wires:
  G/1 -> Add1/2, Add/2, MATLAB Function/1(G)
  X_body/1 -> Cross Product1/2, MATLAB Function/2(vorbit), Cross Product/2
  MATLAB Function/1(yy) -> Product/1
  Zsh/1 -> Abs/1
  Abs/1 -> Product2/3, Product/2
  Constant/1 -> Add/1
  Constant1/1 -> Add1/1
  Add/1 -> Cross Product/1
  Add1/1 -> Cross Product1/1
  Cross Product/1 -> Product1/1
  Constant3/1 -> Product1/2
  Ysh/1 -> Abs1/1
  Abs1/1 -> Product1/3
  Cross Product1/1 -> Product2/1
  Constant2/1 -> Product2/2
  Product1/1 -> Add2/1
  Product2/1 -> Add2/2
  Add2/1 -> Add3/1
  Product/1 -> Add3/2
  Add3/1 -> Product3/1
  velocity/1 -> Product3/2
  density/1 -> Product3/3
  Product3/1 -> Scope/1, Out1/1
  Constant4/1 -> Product3/4
  Constant5/1 -> Product3/5

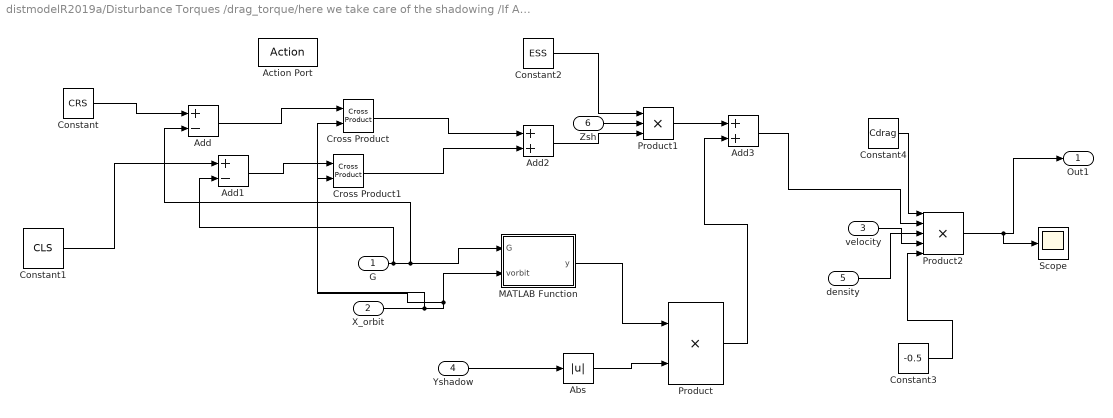
== system distmodelR2019a/Disturbance Torques /drag_torque/here we take care of the shadowing /If Action Subsystem3 ==
  G : Inport
  X_orbit : Inport  Port=2
  velocity : Inport  Port=3
  Yshadow : Inport  Port=4
  density : Inport  Port=5
  Zsh : Inport  Port=6
  Action Port : ActionPort  ActionPortLabel=elseif(u1>0.01&u2<-0.01)
  Abs : Abs
  Add : Sum  Inputs=+-
  Add1 : Sum  Inputs=+-
  Add2 : Sum
  Add3 : Sum
  Constant : Constant  Value=CRS
  Constant1 : Constant  Value=CLS  VectorParams1D=off  SampleTime=-1
  Constant2 : Constant  Value=ESS
  Constant3 : Constant  Value=-0.5
  Constant4 : Constant  Value=Cdrag
  Cross Product : vrlib/Utilities/Cross Product
  Cross Product1 : vrlib/Utilities/Cross Product
  MATLAB Function : MATLAB Function  TreatAsAtomicUnit=on
  Product : Product
  Product1 : Product  Inputs=3
  Product2 : Product  Inputs=5
  Scope : Scope
  Out1 : Outport  VectorParamsAs1DForOutWhenUnconnected=off
  wires:
  MATLAB Function/1(y) -> Product/1
  G/1 -> Add1/2, Add/2, MATLAB Function/1(G)
  Abs/1 -> Product/2
  Yshadow/1 -> Abs/1
  Constant/1 -> Add/1
  Add/1 -> Cross Product/1
  X_orbit/1 -> Cross Product1/2, Cross Product/2, MATLAB Function/2(vorbit)
  Constant1/1 -> Add1/1
  Add1/1 -> Cross Product1/1
  Cross Product1/1 -> Add2/2
  Cross Product/1 -> Add2/1
  Add2/1 -> Product1/3
  Constant2/1 -> Product1/1
  Zsh/1 -> Product1/2
  Product1/1 -> Add3/1
  Product/1 -> Add3/2
  Add3/1 -> Product2/2
  velocity/1 -> Product2/4
  density/1 -> Product2/3
  Product2/1 -> Scope/1, Out1/1
  Constant3/1 -> Product2/5
  Constant4/1 -> Product2/1

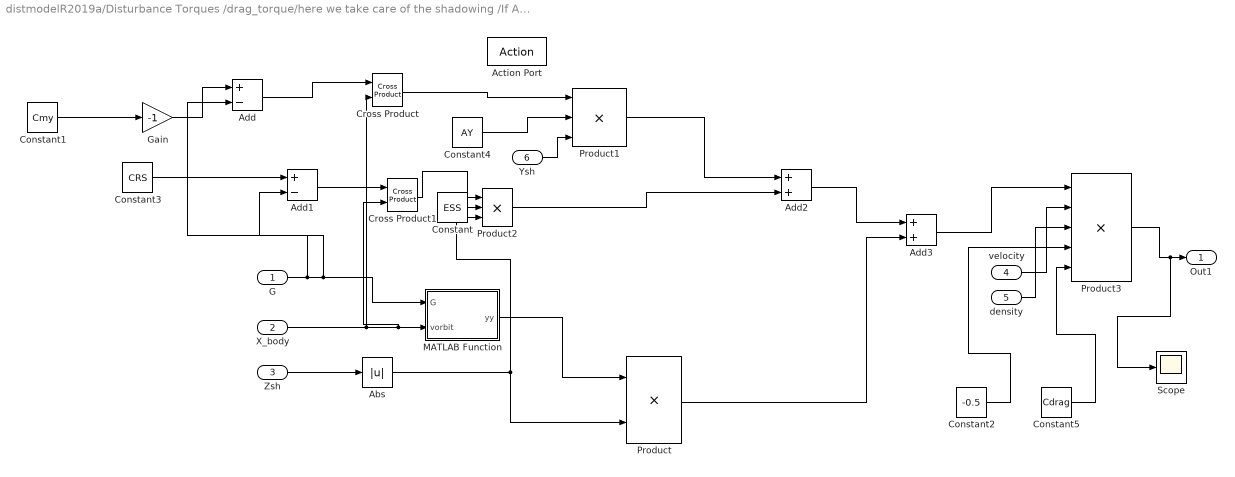
== system distmodelR2019a/Disturbance Torques /drag_torque/here we take care of the shadowing /If Action Subsystem4 ==
  G : Inport
  X_body : Inport  Port=2
  Zsh : Inport  Port=3
  velocity : Inport  Port=4
  density : Inport  Port=5
  Ysh : Inport  Port=6
  Action Port : ActionPort  ActionPortLabel=elseif(u1<-0.01&u2>0.01)
  Abs : Abs
  Add : Sum  Inputs=+-
  Add1 : Sum  Inputs=+-
  Add2 : Sum
  Add3 : Sum
  Constant : Constant  Value=ESS
  Constant1 : Constant  Value=Cmy
  Constant2 : Constant  Value=-0.5
  Constant3 : Constant  Value=CRS
  Constant4 : Constant  Value=AY
  Constant5 : Constant  Value=Cdrag
  Cross Product : vrlib/Utilities/Cross Product
  Cross Product1 : vrlib/Utilities/Cross Product
  Gain : Gain  Gain=-1
  MATLAB Function : MATLAB Function  TreatAsAtomicUnit=on
  Product : Product
  Product1 : Product  Inputs=3
  Product2 : Product  Inputs=3
  Product3 : Product  Inputs=5
  Scope : Scope
  Out1 : Outport  VectorParamsAs1DForOutWhenUnconnected=off
  wires:
  Abs/1 -> Product2/3, Product/2
  Zsh/1 -> Abs/1
  MATLAB Function/1(yy) -> Product/1
  G/1 -> Add/2, Add1/2, MATLAB Function/1(G)
  Constant1/1 -> Gain/1
  Gain/1 -> Add/1
  Constant3/1 -> Add1/1
  Add/1 -> Cross Product/1
  X_body/1 -> Cross Product/2, Cross Product1/2, MATLAB Function/2(vorbit)
  Cross Product/1 -> Product1/1
  Constant4/1 -> Product1/2
  Ysh/1 -> Product1/3
  Add1/1 -> Cross Product1/1
  Cross Product1/1 -> Product2/1
  Constant/1 -> Product2/2
  Product2/1 -> Add2/2
  Product1/1 -> Add2/1
  Add2/1 -> Add3/1
  Product/1 -> Add3/2
  Add3/1 -> Product3/1
  velocity/1 -> Product3/2
  density/1 -> Product3/3
  Product3/1 -> Scope/1, Out1/1
  Constant2/1 -> Product3/4
  Constant5/1 -> Product3/5

== system distmodelR2019a/resudial mgnetique torque /IGRF Computation block/Obtain B_ECI/Dipole Subsystem ==
  In1 : Inport
  Action Port : ActionPort  ActionPortLabel=else
  Bus Selector1 : BusSelector  OutputSignals=h,lat,long,DCM_i2e
  Dipole Model : Subsystem  AncestorBlock=DipoleModel/Dipole Model
  "B_ECI " : Outport  VectorParamsAs1DForOutWhenUnconnected=off
  wires:
  In1/1 -> Bus Selector1/1
  Bus Selector1/1 -> Dipole Model/1(h)  "<h>"
  Bus Selector1/2 -> Dipole Model/2("lat ")  "<lat>"
  Bus Selector1/3 -> Dipole Model/3(long)  "<long>"
  Bus Selector1/4 -> Dipole Model/4(ECI2ECEF_DCM)  "<DCM_i2e>"
  Dipole Model/1("B_ECI ") -> "B_ECI "/1

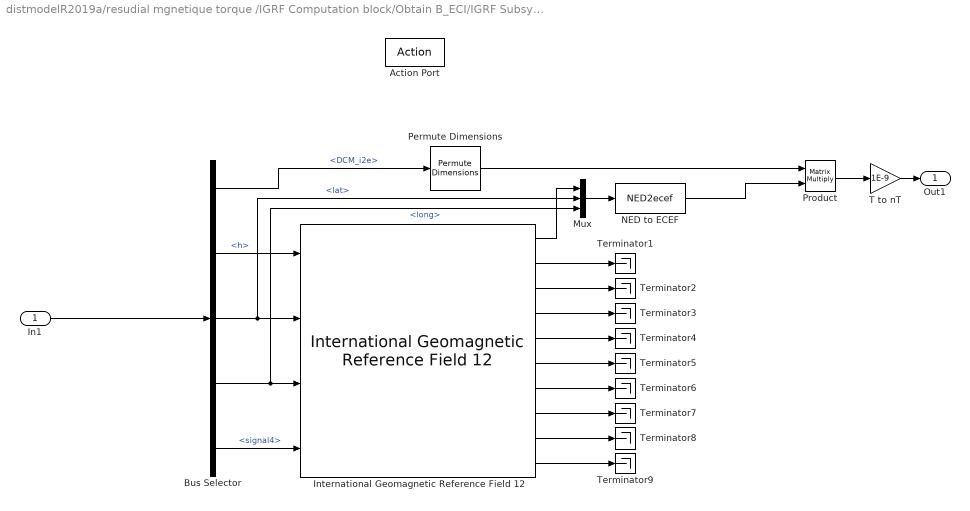
== system distmodelR2019a/resudial mgnetique torque /IGRF Computation block/Obtain B_ECI/IGRF Subsystem ==
  In1 : Inport
  Action Port : ActionPort  ActionPortLabel=if(u1 > 0)
  Bus Selector : BusSelector  OutputSignals=DCM_i2e,h,lat,long,signal4
  International Geomagnetic Reference Field 12 : aerolibobsolete/International Geomagnetic Reference Field 12  units=Metric (MKS)  time_in=on  month=January  day=1  year=2020  action=None  sv_out=on
      settings: SourceProductBaseCode=AE
  Mux : Mux  Inputs=3
  NED to ECEF : MATLABFcn  MATLABFcn=NED2ecef  OutputDimensions=[3;1]  Output1D=off
  Permute Dimensions : PermuteDimensions
  Product : Product  Multiplication=Matrix(*)
  T to nT : Gain  Gain=1E-9
  Terminator{1..9} (9 alike) : Terminator
  Out1 : Outport  VectorParamsAs1DForOutWhenUnconnected=off
  wires:
  In1/1 -> Bus Selector/1
  Bus Selector/2 -> International Geomagnetic Reference Field 12/1  "<h>"
  T to nT/1 -> Out1/1
  Bus Selector/5 -> International Geomagnetic Reference Field 12/4  "<signal4>"
  Bus Selector/4 -> Mux/3, International Geomagnetic Reference Field 12/3  "<long>"
  Bus Selector/3 -> Mux/2, International Geomagnetic Reference Field 12/2  "<lat>"
  International Geomagnetic Reference Field 12/2 -> Terminator1/1
  International Geomagnetic Reference Field 12/10 -> Terminator9/1
  International Geomagnetic Reference Field 12/4 -> Terminator3/1
  International Geomagnetic Reference Field 12/5 -> Terminator4/1
  International Geomagnetic Reference Field 12/3 -> Terminator2/1
  International Geomagnetic Reference Field 12/1 -> Mux/1
  International Geomagnetic Reference Field 12/6 -> Terminator5/1
  International Geomagnetic Reference Field 12/8 -> Terminator7/1
  International Geomagnetic Reference Field 12/7 -> Terminator6/1
  International Geomagnetic Reference Field 12/9 -> Terminator8/1
  Bus Selector/1 -> Permute Dimensions/1  "<DCM_i2e>"
  Permute Dimensions/1 -> Product/1
  Product/1 -> T to nT/1
  Mux/1 -> NED to ECEF/1
  NED to ECEF/1 -> Product/2

== system distmodelR2019a/resudial mgnetique torque /IGRF Computation block/Obtain B_ECI/Dipole Subsystem/Dipole Model ==
  h : Inport
  "lat " : Inport  Port=2
  long : Inport  Port=3
  ECI2ECEF_DCM : Inport  Port=4
  Bus Creator : BusCreator  Inputs=3
  Interpreted MATLAB Function : MATLABFcn  MATLABFcn=DipoleMod(u(1),u(2),u(3),nmax)
  Permute Dimensions : PermuteDimensions
  Product : Product  Multiplication=Matrix(*)
  scaling from nT to T : Gain  Gain=1e-9
  "B_ECI " : Outport  VectorParamsAs1DForOutWhenUnconnected=off
  wires:
  Product/1 -> scaling from nT to T/1
  Permute Dimensions/1 -> Product/1
  ECI2ECEF_DCM/1 -> Permute Dimensions/1
  Bus Creator/1 -> Interpreted MATLAB Function/1
  "lat "/1 -> Bus Creator/2
  long/1 -> Bus Creator/3
  scaling from nT to T/1 -> "B_ECI "/1
  Interpreted MATLAB Function/1 -> Product/2
  h/1 -> Bus Creator/1

== matlab function distmodelR2019a/resudial mgnetique torque /IGRF Computation block/ECI To LLA ==
  data: X_ECEF input; h output; lat output; long output
function [h, lat, long] = fcn(X_ECEF)
    h = 0;
    lat = 0;
    long = 0;
[lat, long, h] = ecef2geod(X_ECEF(1),X_ECEF(2),X_ECEF(3));

== matlab function distmodelR2019a/Disturbance Torques /drag_torque/here we take care of the shadowing /If Action Subsystem/MATLAB Function ==
  data: G input; vorbit input; y output
function y = fcn(G, vorbit)
% les 4 points qui delimite le cadre 1
A=[0.17,0.11,0.05];%ok
B=[0.17,0.28,0.05];
C=[-0.17,0.28,0.05];
D=[-0.17,0.11,0.05];%ok


torque=[0,0,0];


%projection of B
pBy=0.11;
t=(pBy-B(2))/vorbit(2);
pBx=B(1)+t*vorbit(1);
pBz=B(3)+t*vorbit(3);

%projection of c
pCy=pBy;
pCx=C(1)+t*vorbit(1);%% because they have the same y
pCz=pBz;%%because of //
%vecteur directeur de notre droite
ux=A(1)-pBx;
uy=A(2)-pBy;%% zero we are in zx plan
uz=A(3)-pBz;
if pCz>-0.05
    if pBx<0.17
        
        if pBx>-0.17 %%we caculate(frcement pCx<-0.17)
            %pas
            N=100;%%%%%%%%%%%%%%%%%%%can be changed
            pas=ux/N;
            %integrale de rieman
            for i=0:N-1
                x=pBx+i*pas;
                t=(x-A(1))/ux;
                z=A(3)+t*uz;
                %geometric center for dA
                Gc=[x+(pas/2),pBy,(z-0.05)/2];
                Rs=Gc-G;
                torque= torque +cross(Rs,vorbit)*((z+0.05)*pas);
            end
            %the other surface
            Gc=[(pBx-0.17)/2,pBy,(pBz-0.05)/2];
            Rs=Gc-G;
            torque=torque+(pBx+0.17)*(pBz+0.05)*cross(Rs,vorbit);
        else
            %%we starte (la droite (ApB) coupe [segment]
            N=200;
            pas=0.34/N;
            
            for i=0:N-1
                x=-0.17+i*pas;
                t=(x-A(1))/ux;
                z=A(3)+t*uz;
                Gc=[x+(pas/2),pBy,(z-0.05)/2];
                Rs=Gc-G;
                torque= torque +cross(Rs,vorbit)*((z+0.05)*pas);
                
            end
            
            
            
        end
        
    elseif pCx<0.17 %%we konw already that pCx>-0.17
        %we calculate
        ux=D(1)-pCx;
        uy=D(2)-pCy;%%zero
        uz=D(3)-pCz;
        N=100;
        pas=ux/N;%negative always
       
        for i=0:N-1
            x=pCx+i*pas;
            t=(x-D(1))/ux;
            z=D(3)+t*uz;
            %geometric center for dA
            Gc=[x+(pas/2),pCy,(z-0.05)/2];
            Rs=Gc-G;
            torque= torque +cross(Rs,vorbit)*((z+0.05)*pas);
            
        end
        Gc=[(pCx+0.17)/2,pCy,(pCz-0.05)/2];
        Rs=Gc-G;
        torque=torque+(0.17-pCx)*(pCz+0.05)*cross(Rs,vorbit);
    else
        ux=D(1)-pCx;
        uy=D(2)-pCy;
        uz=D(3)-pCz;
        %we calculate(coupe droite segment)
        N=200;
        pas=-0.34/N;
     
        for i=0:N-1
            x=0.17+i*pas;
            t=(x-D(1))/ux;
            z=D(3)+t*uz;
            Gc=[x+(pas/2),pCy,(z-0.05)/2];
            Rs=Gc-G;
            torque= torque +cross(Rs,vorbit)*((z+0.05)*pas);
            
        end
        
    end
else
    %let Dprim Aprim to be like
    Dprim=[-0.17,0.11,-0.05];
    Aprim=[0.17,0.11,-0.05];
    if pBx<0.17
        ux=A(1)-pBx;
        uy=A(2)-pBy;
        uz=A(3)-pBz;
        %%%%
        ADpv=A-Dprim;
        %%%%%
        tprim=(pBz-A(3))/ADpv(3);
        %on compare
        xc=A(1)+tprim*ADpv(1);
        if pBx<xc%%%derriere suivant les x negative
            N=200;%%%%%%%%%%%%%%%%%%%can be changed
            pas=0.34/N;
            %integrale de rieman
            
            for i=0:N-1
                x=-0.17+i*pas;%%%intersection DDprim
                t=(x-A(1))/ux;
                z=A(3)+t*uz;
                %geometric center for dA
                Gc=[x+(pas/2),pBy,(z-0.05)/2];
                Rs=Gc-G;
                torque= torque +cross(Rs,vorbit)*((z+0.05)*pas);
            end
            
        else
            %we calculate%%%%%%%%%%problem(we can use diagonale)
            t=(-0.05-A(3))/uz;%%intersection DprimAprim
            x=A(1)+t*ux;
            N=100;%%%%%%%%%%%%%%%%%%%can be changed
            pas=(0.17-x)/N;
            %integrale de rieman
          
            for i=0:N-1
                x=x+i*pas;
                t=(x-A(1))/ux;
                z=A(3)+t*uz;
                %geometric center for dA
                Gc=[x+(pas/2),pBy,(z-0.05)/2];
                Rs=Gc-G;
                torque= torque +cross(Rs,vorbit)*((z+0.05)*pas);
            end
            
            
            
        end
        %%elseif pCx<0.17
        %we calculate
    else
        ux=D(1)-pCx;
        uy=D(2)-pCy;
        uz=D(3)-pCz;
        %%%%
        DApv=D-Aprim;
        %%%%%
        tprim=(pCz-A(3))/DApv(3);
        %on compare
        xc=D(1)+tprim*DApv(1);
        
        if pCx>xc
            N=200;%%%%%%%%%%%%%%%%%%%can be changed
            pas=-0.34/N;
            %integrale de rieman
            
            for i=0:N-1
                x=0.17+i*pas;
                t=(x-D(1))/ux;
                z=D(3)+t*uz;
                %geometric center for dA
                Gc=[x+(pas/2),pCy,(z-0.05)/2];
                Rs=Gc-G;
                torque= torque +cross(Rs,vorbit)*((z+0.05)*pas);
            end
            
        else
            %we calculate%%%%%%%%%%problem(we can use diagonale)
            t=(-0.05-D(3))/uz;
            x=D(1)+t*ux;
            N=100;%%%%%%%%%%%%%%%%%%%can be changed
            pas=(-0.17-x)/N;
            %integrale de rieman
           
            for i=0:N-1
                x=x+i*pas;
                t=(x-D(1))/ux;
                z=D(3)+t*uz;
                %geometric center for dA
                Gc=[x+(pas/2),pBy,(z-0.05)/2];
                Rs=Gc-G;
                torque= torque +cross(Rs,vorbit)*((z+0.05)*pas);
            end
            
            
            
        end
        
    end
    
end

y = torque;

== matlab function distmodelR2019a/Disturbance Torques /MATLAB Function2 ==
  data: u input; y output
function y = fcn(u)
y = u(6);

== matlab function distmodelR2019a/Time propagator/UTC to JD ==
  data: Time_UTC input; JD output
function JD = fcn(Time_UTC)

% JD = juliandate(Time_UTC);
JD = Dt2jD(Time_UTC);

== matlab function distmodelR2019a/Time propagator/JD to UTC ==
  data: JD input; Time_UTC output
function Time_UTC = fcn(JD)
    coder.extrinsic('datetime','datevec');
    Time_UTC = [0,0,0,0,0,0];
Time_UTC =  datevec(datetime(JD,'convertfrom','juliandate'));
